simulink model "single_robot_control"  (R2020a)
settings: Solver=FixedStepAuto  StartTime=0.0  StopTime=10  RelTol=1e-3
settings Model: Creator=sanim  LastModifiedBy=Dell
settings DataIOCC: ReturnWorkspaceOutputs=off
settings DebuggingCC: ArithmeticOperatorsInVariantConditions=warning
settings SFSimCC: CustomCodeUndefinedFunction=UseInterfaceOnly

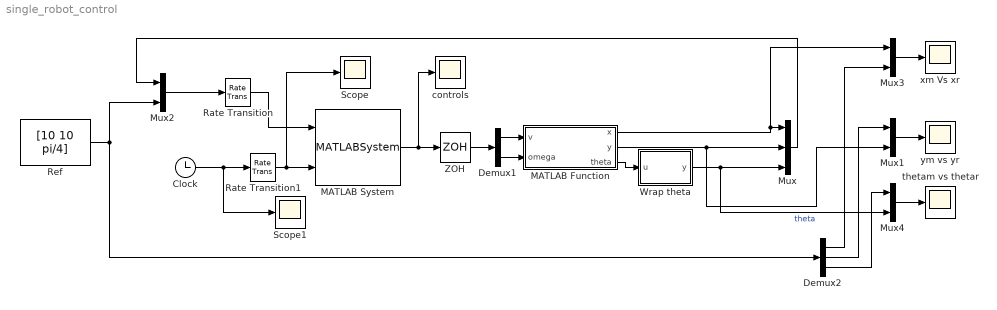
== system single_robot_control ==
  Clock : Clock
  Demux1 : Demux  Outputs=2
  Demux2 : Demux  Outputs=3
  MATLAB Function : MATLAB Function  TreatAsAtomicUnit=on
  MATLAB System : MATLABSystem  System=controller  SimulateUsing=Interpreted execution
      mask Type: controller
      mask Display:
      | disp('controller');
      | port_label('input',1,'x');
      | port_label('input',2,'t');
      | port_label('output',1,'u');
  Mux : Mux  Inputs=3
  Mux{1..4} (4 alike) : Mux  Inputs=2
  Rate Transition : RateTransition  OutPortSampleTime=0.01
  Rate Transition1 : RateTransition  OutPortSampleTime=0.01
  Ref : Constant  Value=[10 10 pi/4]
  Scope : Scope
  Scope1 : Scope
  Wrap theta : MATLAB Function  TreatAsAtomicUnit=on
  ZOH : ZeroOrderHold  SampleTime=0.05
  controls : Scope
  thetam vs thetar : Scope
  xm Vs xr : Scope
  ym vs yr : Scope
  wires:
  MATLAB Function/2(y) -> Mux1/2, Mux/2
  ZOH/1 -> Demux1/1
  Mux/1 -> Mux2/1
  Ref/1 -> Demux2/1, Mux2/2
  Rate Transition/1 -> MATLAB System/1
  MATLAB System/1 -> ZOH/1, controls/1
  Demux1/1 -> MATLAB Function/1(v)
  MATLAB Function/1(x) -> Mux3/1, Mux/1
  Rate Transition1/1 -> Scope/1, MATLAB System/2
  Demux1/2 -> MATLAB Function/2(omega)
  Clock/1 -> Scope1/1, Rate Transition1/1
  Mux2/1 -> Rate Transition/1
  Demux2/1 -> Mux3/2
  Mux3/1 -> xm Vs xr/1
  Demux2/2 -> Mux1/1
  Mux1/1 -> ym vs yr/1
  Mux4/1 -> thetam vs thetar/1
  Demux2/3 -> Mux4/1
  MATLAB Function/3(theta) -> Wrap theta/1(u)
  Wrap theta/1(y) -> Mux4/2, Mux/3  "theta"

== matlab function single_robot_control/MATLAB Function ==
  data: v input; x output; omega input; y output; theta output
function [x,y,theta]= rhs(v,omega)
persistent x_dotP y_dotP omegaP
V0=0;
x0=2;
y0=1;
theta0=0;
if isempty(omegaP)
    omegaP=0;
    x_dotP=0;
    y_dotP=0;
end
omega1= omega+omegaP;
theta = omega1+ theta0;
x_dot=(v+V0)*(cos(theta));
y_dot=(v+V0)*(sin(theta));
x_dot1=x_dot+x_dotP;
y_dot1=y_dot+y_dotP;
x=x_dot1+x0;
y=y_dot1+y0;
omegaP=omega1;
x_dotP=x_dot1;
y_dotP=y_dot1;
end

== matlab function single_robot_control/Wrap theta ==
  data: u input; y output
function y = Theta(u)
%#codegen

positiveInput = (u > 0);
y = mod(u, 2*pi);
y((u == 0) & positiveInput) = 2*pi;
